simulink model "LogicalAND4bit"  (R2025b)
settings: Solver=VariableStepAuto  StartTime=0.0  StopTime=10.0  RelTol=1e-3
settings Model: Creator=cyber  LastModifiedBy=cyber

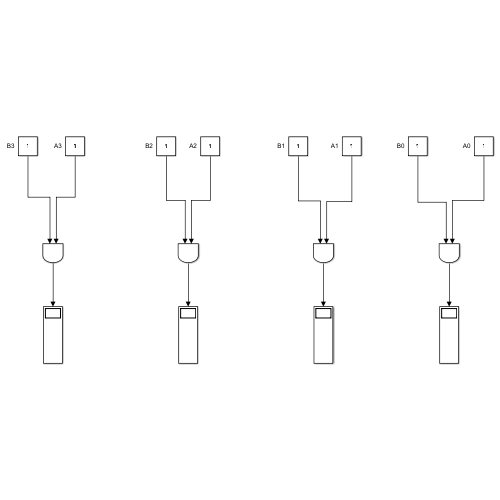
[thumbnail: Simulink's stored preview of the top-level diagram]
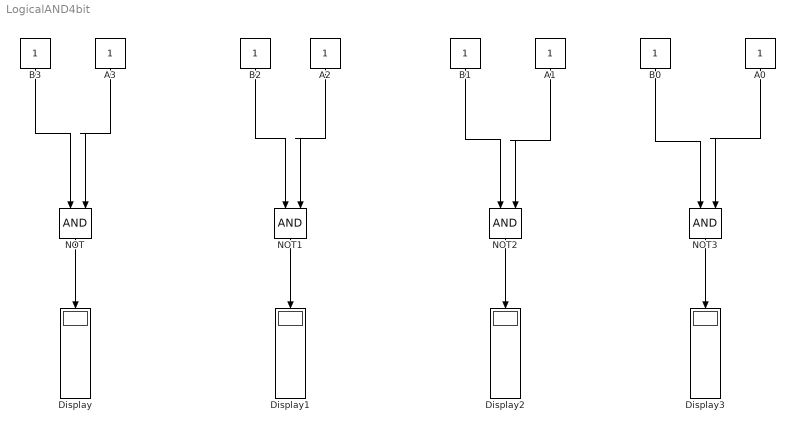
== system LogicalAND4bit ==
  A{0..3} (4 alike) : Constant
  B{0..3} (4 alike) : Constant
  Display{,1..3} (4 alike) : Display
  NOT{,1..3} (4 alike) : Logic  IconShape=distinctive  AllPortsSameDT=off  OutDataTypeStr=boolean
  wires:
  B3/1 -> NOT/1
  A3/1 -> NOT/2
  B2/1 -> NOT1/1
  A2/1 -> NOT1/2
  B1/1 -> NOT2/1
  A1/1 -> NOT2/2
  B0/1 -> NOT3/1
  A0/1 -> NOT3/2
  NOT1/1 -> Display1/1
  NOT/1 -> Display/1
  NOT2/1 -> Display2/1
  NOT3/1 -> Display3/1
